simulink model "OMAP"  (R2018b)
settings: Solver=FixedStepDiscrete  StartTime=0.0  StopTime=10.0  FixedStep=0.01  RelTol=1e-3
values from neighbouring files (symbols this model uses):
  Clb_ICADirect_LaneDisp_StateFive = Simulink.Parameter    [omap_ver_442.m]
  Clb_ICADirect_LaneDisp_StateFour = Simulink.Parameter    [omap_ver_442.m]
  Clb_ICADirect_LaneDisp_StateOne = Simulink.Parameter    [omap_ver_442.m]
  Clb_ICADirect_LaneDisp_StateThree = Simulink.Parameter    [omap_ver_442.m]
  Clb_ICADirect_LaneDisp_StateTwo = Simulink.Parameter    [omap_ver_442.m]
  Clb_ICADirect_LaneDisp_StateZero = Simulink.Parameter    [omap_ver_442.m]
  Clb_ICADirect_LaneDispSW = Simulink.Parameter    [omap_ver_442.m]
  Clb_ICADirect_TrnLghtsCom_Switch = Simulink.Parameter    [omap_ver_442.m]
  Clb_ICADirect_TrnLghtsCom_Value = Simulink.Parameter    [omap_ver_442.m]
  Clb_ICADirect_TrnLghtsCrtl_Inhb = Simulink.Parameter    [omap_ver_442.m]
  OMAP_ACCAEB_EMSESC_Decel = Simulink.Parameter    [omap_ver_442.m]
  OMAP_ACCFCW_IC_Decel = Simulink.Parameter    [omap_ver_442.m]
  OMAP_clb_ACC_RVVReqType = Simulink.Parameter    [omap_ver_442.m]
  OMAP_clb_ACC_RVVReqType_Switch = Simulink.Parameter    [omap_ver_442.m]
  OMAP_clb_ACCHeadwayDisplay = Simulink.Parameter    [omap_ver_442.m]
  OMAP_clb_ACCHeadwayDisplay_Switch = Simulink.Parameter    [omap_ver_442.m]
  OMAP_clb_ACCHeadwayIcon = Simulink.Parameter    [omap_ver_442.m]
  OMAP_clb_ACCHeadwayIcon_Switch = Simulink.Parameter    [omap_ver_442.m]
  OMAP_clb_ACCMessagePrompt = Simulink.Parameter    [omap_ver_442.m]
  OMAP_clb_ACCMessagePrompt_Switch = Simulink.Parameter    [omap_ver_442.m]
  OMAP_clb_ACCRequestEPB = Simulink.Parameter    [omap_ver_442.m]
  OMAP_clb_ACCRequestEPB_Switch = Simulink.Parameter    [omap_ver_442.m]
  OMAP_clb_ACCSetSpeed = Simulink.Parameter    [omap_ver_442.m]
  OMAP_clb_ACCSetSpeed_Switch = Simulink.Parameter    [omap_ver_442.m]
  OMAP_clb_ACCSetSpeedDis = Simulink.Parameter    [omap_ver_442.m]
  OMAP_clb_ACCSetSpeedDis_Switch = Simulink.Parameter    [omap_ver_442.m]
  OMAP_clb_ACCState = Simulink.Parameter    [omap_ver_442.m]
  OMAP_clb_ACCState_Switch = Simulink.Parameter    [omap_ver_442.m]
  OMAP_clb_ACCStatusIconDis = Simulink.Parameter    [omap_ver_442.m]
  OMAP_clb_ACCStatusIconDis_Switch = Simulink.Parameter    [omap_ver_442.m]
  OMAP_clb_ACCTorqueReq = Simulink.Parameter    [omap_ver_442.m]
  OMAP_clb_ACCTorqueReq_Switch = Simulink.Parameter    [omap_ver_442.m]
  OMAP_clb_ADAS_State = Simulink.Parameter    [omap_ver_442.m]
  OMAP_clb_ADAS_State_Switch = Simulink.Parameter    [omap_ver_442.m]
  OMAP_clb_AEBAlertReq = Simulink.Parameter    [omap_ver_442.m]
  OMAP_clb_AEBAlertReq_Switch = Simulink.Parameter    [omap_ver_442.m]
  OMAP_clb_AEBBrakingProg = Simulink.Parameter    [omap_ver_442.m]
  OMAP_clb_AEBBrakingProg_Switch = Simulink.Parameter    [omap_ver_442.m]
  OMAP_clb_AEBFaultStatus = Simulink.Parameter    [omap_ver_442.m]
  OMAP_clb_AEBFaultStatus_Switch = Simulink.Parameter    [omap_ver_442.m]
  OMAP_clb_AEBMassageDisp = Simulink.Parameter    [omap_ver_442.m]
  OMAP_clb_AEBMassageDisp_Switch = Simulink.Parameter    [omap_ver_442.m]
  OMAP_clb_AEBState = Simulink.Parameter    [omap_ver_442.m]
  OMAP_clb_AEBState_Switch = Simulink.Parameter    [omap_ver_442.m]
  OMAP_clb_AEBSwitchStatus = Simulink.Parameter    [omap_ver_442.m]
  OMAP_clb_AEBSwitchStatus_Switch = Simulink.Parameter    [omap_ver_442.m]
  OMAP_clb_BrakeRequest = Simulink.Parameter    [omap_ver_442.m]
  OMAP_clb_BrakeRequest_Switch = Simulink.Parameter    [omap_ver_442.m]
  OMAP_clb_DecelerationSet = Simulink.Parameter    [omap_ver_442.m]
  OMAP_clb_DecelerationSet_Switch = Simulink.Parameter    [omap_ver_442.m]
  OMAP_clb_DecelerationType = Simulink.Parameter    [omap_ver_442.m]
  OMAP_clb_DecelerationType_Switch = Simulink.Parameter    [omap_ver_442.m]
  OMAP_clb_DeclControlReq = Simulink.Parameter    [omap_ver_442.m]
  OMAP_clb_DeclControlReq_Switch = Simulink.Parameter    [omap_ver_442.m]
  OMAP_clb_DownorUpGearMinTime = Simulink.Parameter    [omap_ver_442.m]
  OMAP_clb_DownorUpGearMinTime_Switch = Simulink.Parameter    [omap_ver_442.m]
  OMAP_clb_ELKPopupMessage = Simulink.Parameter    [omap_ver_442.m]
  OMAP_clb_ELKPopupMessage_Switch = Simulink.Parameter    [omap_ver_442.m]
  OMAP_clb_ELKSts = Simulink.Parameter    [omap_ver_442.m]
  OMAP_clb_ELKSts_Switch = Simulink.Parameter    [omap_ver_442.m]
  OMAP_clb_ESAFaultSt = Simulink.Parameter    [omap_ver_442.m]
  OMAP_clb_ESAFaultSt_Switch = Simulink.Parameter    [omap_ver_442.m]
  OMAP_clb_ESARequest = Simulink.Parameter    [omap_ver_442.m]
  OMAP_clb_ESARequest_Switch = Simulink.Parameter    [omap_ver_442.m]
  OMAP_clb_ESAState = Simulink.Parameter    [omap_ver_442.m]
  OMAP_clb_ESAState_Switch = Simulink.Parameter    [omap_ver_442.m]
  OMAP_clb_ESATorqueReq = Simulink.Parameter    [omap_ver_442.m]
  OMAP_clb_ESATorqueReq_Switch = Simulink.Parameter    [omap_ver_442.m]
  OMAP_clb_ESCDriveOff = Simulink.Parameter    [omap_ver_442.m]
  OMAP_clb_ESCDriveOff_Switch = Simulink.Parameter    [omap_ver_442.m]
  OMAP_clb_ESCHoldReq = Simulink.Parameter    [omap_ver_442.m]
  OMAP_clb_ESCHoldReq_Switch = Simulink.Parameter    [omap_ver_442.m]
  OMAP_clb_Handsoffwarning = Simulink.Parameter    [omap_ver_442.m]
  OMAP_clb_Handsoffwarning_Switch = Simulink.Parameter    [omap_ver_442.m]
  OMAP_clb_HapticAlarmReq = Simulink.Parameter    [omap_ver_442.m]
  OMAP_clb_HapticAlarmReq_Switch = Simulink.Parameter    [omap_ver_442.m]
  OMAP_clb_HMIPopupMassage = Simulink.Parameter    [omap_ver_442.m]
  OMAP_clb_HMIPopupMassage_Switch = Simulink.Parameter    [omap_ver_442.m]
  OMAP_clb_HWAActionSts = Simulink.Parameter    [omap_ver_442.m]
  OMAP_clb_HWAActionSts_Switch = Simulink.Parameter    [omap_ver_442.m]
  OMAP_clb_HWAMode = Simulink.Parameter    [omap_ver_442.m]
  OMAP_clb_HWAMode_Switch = Simulink.Parameter    [omap_ver_442.m]
  OMAP_clb_HWATurnOnIdctr = Simulink.Parameter    [omap_ver_442.m]
  OMAP_clb_HWATurnOnIdctr_Switch = Simulink.Parameter    [omap_ver_442.m]
  OMAP_clb_ICAMassageDisp = Simulink.Parameter    [omap_ver_442.m]
  OMAP_clb_ICAMassageDisp_Switch = Simulink.Parameter    [omap_ver_442.m]
  OMAP_clb_ICAStatusIcon = Simulink.Parameter    [omap_ver_442.m]
  OMAP_clb_ICAStatusIcon_Switch = Simulink.Parameter    [omap_ver_442.m]
  OMAP_clb_ISLCDriverRemind = Simulink.Parameter    [omap_ver_442.m]
  OMAP_clb_ISLCDriverRemind_Switch = Simulink.Parameter    [omap_ver_442.m]
  OMAP_clb_ISLCState = Simulink.Parameter    [omap_ver_442.m]
  OMAP_clb_ISLCState_Switch = Simulink.Parameter    [omap_ver_442.m]
  OMAP_clb_JAFaultSt = Simulink.Parameter    [omap_ver_442.m]
  OMAP_clb_JAFaultSt_Switch = Simulink.Parameter    [omap_ver_442.m]
  OMAP_clb_LCAPopupMessage = Simulink.Parameter    [omap_ver_442.m]
  OMAP_clb_LCAPopupMessage_Switch = Simulink.Parameter    [omap_ver_442.m]
  OMAP_clb_LCAStatusDisplay = Simulink.Parameter    [omap_ver_442.m]
  OMAP_clb_LCAStatusDisplay_Switch = Simulink.Parameter    [omap_ver_442.m]
  OMAP_clb_LDWStatusDisplay = Simulink.Parameter    [omap_ver_442.m]
  OMAP_clb_LDWStatusDisplay_Switch = Simulink.Parameter    [omap_ver_442.m]
  OMAP_clb_LDWWarningSt = Simulink.Parameter    [omap_ver_442.m]
  OMAP_clb_LDWWarningSt_Switch = Simulink.Parameter    [omap_ver_442.m]
  OMAP_clb_LightControlValid = Simulink.Parameter    [omap_ver_442.m]
  OMAP_clb_LightControlValid_Switch = Simulink.Parameter    [omap_ver_442.m]
  OMAP_clb_LKAActivation = Simulink.Parameter    [omap_ver_442.m]
  OMAP_clb_LKAActivation_Switch = Simulink.Parameter    [omap_ver_442.m]
  OMAP_clb_LKAAngleReq = Simulink.Parameter    [omap_ver_442.m]
  OMAP_clb_LKAAngleReq_Switch = Simulink.Parameter    [omap_ver_442.m]
  OMAP_clb_LKAMode = Simulink.Parameter    [omap_ver_442.m]
  OMAP_clb_LKAMode_Switch = Simulink.Parameter    [omap_ver_442.m]
  OMAP_clb_LKAorELK_CoolTime = Simulink.Parameter    [omap_ver_442.m]
  OMAP_clb_LKAState = Simulink.Parameter    [omap_ver_442.m]
  OMAP_clb_LKAState_Switch = Simulink.Parameter    [omap_ver_442.m]
  OMAP_clb_LKAStatusDisplay = Simulink.Parameter    [omap_ver_442.m]
  OMAP_clb_LKAStatusDisplay_Switch = Simulink.Parameter    [omap_ver_442.m]
  OMAP_clb_LKASwitchState = Simulink.Parameter    [omap_ver_442.m]
  OMAP_clb_LKASwitchState_Switch = Simulink.Parameter    [omap_ver_442.m]
  OMAP_clb_LKATorqFactReq = Simulink.Parameter    [omap_ver_442.m]
  OMAP_clb_LKATorqFactReq_Switch = Simulink.Parameter    [omap_ver_442.m]
  OMAP_clb_PrefillRequest = Simulink.Parameter    [omap_ver_442.m]
  ... (+36 more)
libraries: simulink x184, canmsglib x2
(part 9 of 14)

== system OMAP/Runnable_OMAP_10ms_sys/OMAP_Module/Subsystem/ESC_Arbitration/ACC//ICA_arb_AEB//JA ==
  note: 仲裁#3——ACC/ICA与AEB/JAEB
      | 1. 当ACC/ICA在控车且造成的实车减速度已达到（标定值暂定-2.3），若AEB只触发第一档刹车（-2），则仍以ACC/ICA优先。实时监测运算，以当前周期的实车减速度数值为准。
      | 2. 若AEB进一步触发了第二档刹车（-2以上），或者触发了JAEB刹车（总共就一档，-2以上），则AEB/JAEB根据自身的运算正常触发，无条件优先于ACC/ICA
  Input_ACCS : Inport
  Input_AEBS : Inport  Port=2
  Input_JABS : Inport  Port=3
  Input_ELKS : Inport  Port=4
  Input_IMAP : Inport  Port=5
  AEB_arb_JA : Subsystem
  Bus Creator2 : BusCreator  Inputs=8
  Bus Selector : BusSelector  OutputSignals=IMAPve_g_ESC_LonAcc_convert
  Bus Selector4 : BusSelector  OutputSignals=actuator.Function_Acc_status,actuator.OMAPve_y_ADAS_ESCDriveOff,actuator.OMAPve_y_ADAS_ESCHoldReq,actuator.MDD_deceleration_type,actuator.MDD_Decelerationcontrol_request,actuator.Deceleration_setpoint_device,actuator.OMAPve_y_ADAS_ACCRequestEPB
  Compare To Constant : simulink/Logic and Bit Operations/Compare To Constant  relop=>=  const=OMAP_ACCAEB_EMSESC_Decel  OutDataTypeStr=boolean
  Compare To Constant2 : simulink/Logic and Bit Operations/Compare To Constant  relop===  const=4  OutDataTypeStr=boolean
  Compare To Constant3 : simulink/Logic and Bit Operations/Compare To Constant  relop===  const=6  OutDataTypeStr=boolean
  Compare To Constant4 : simulink/Logic and Bit Operations/Compare To Constant  relop=~=  const=4  OutDataTypeStr=boolean
  Compare To Constant5 : simulink/Logic and Bit Operations/Compare To Constant  relop=~=  const=6  OutDataTypeStr=boolean
  Constant : Constant  Value=0  OutDataTypeStr=uint8
  Data Type Conversion1 : DataTypeConversion  OutDataTypeStr=single
  Data Type Conversion{2..5,15,17} (6 alike) : DataTypeConversion  OutDataTypeStr=uint8
  Logical Operator1 : Logic  AllPortsSameDT=off  OutDataTypeStr=boolean
  Logical Operator2 : Logic  Operator=OR  AllPortsSameDT=off  OutDataTypeStr=boolean
  Logical Operator3 : Logic  AllPortsSameDT=off  OutDataTypeStr=boolean
  Logical Operator4 : Logic  Operator=OR  AllPortsSameDT=off  OutDataTypeStr=boolean
  Logical Operator5 : Logic  AllPortsSameDT=off  OutDataTypeStr=boolean
  Switch : Switch  Criteria=u2 ~= 0
  Switch1 : Switch  Criteria=u2 ~= 0
  Out1 : Outport
  Out2 : Outport  Port=2
  tag scope: ob_isJAorDeepAEB=global, ob_isLowACCandLowAEB=global
  wires:
  Switch/1 -> Out2/1
  Data Type Conversion1/1 -> Bus Creator2/7  "OMAPve_g_Deceleration_setpoint_device_1"
  Input_ACCS/1 -> Bus Selector4/1
  Constant/1 -> Bus Creator2/4  "OMAPve_y_AEB_Braking_progress_1"
  Data Type Conversion3/1 -> Bus Creator2/5  "OMAPve_y_Decel_Request_1"
  Bus Selector4/5 -> Data Type Conversion15/1, Data Type Conversion3/1  "<MDD_Decelerationcontrol_request>"
  Data Type Conversion17/1 -> Bus Creator2/3  "OMAPve_y_MDD_deceleration_type_1"
  Data Type Conversion15/1 -> Bus Creator2/6  "OMAPve_y_MDD_Decelerationcontrol_request_1"
  Bus Selector/1 -> Compare To Constant/1  "<IMAPve_g_ESC_LonAcc_convert>"
  Bus Selector4/4 -> Data Type Conversion17/1  "<MDD_deceleration_type>"
  Switch1/1 -> Switch/3
  Bus Creator2/1 -> Switch1/3
  AEB_arb_JA/2(Out2) -> Switch1/1, Switch/1
  Input_AEBS/1 -> AEB_arb_JA/1(Input_AEBS)
  Input_JABS/1 -> AEB_arb_JA/2(Input_JABS)
  AEB_arb_JA/1(Out1) -> Out1/1
  Input_IMAP/1 -> Bus Selector/1
  Logical Operator2/1 -> Logical Operator1/2
  Logical Operator5/1 -> Logical Operator2/1
  Bus Selector4/6 -> Data Type Conversion1/1  "<Deceleration_setpoint_device>"
  Logical Operator3/1 -> Logical Operator2/2
  Logical Operator4/1 -> Logical Operator3/1
  AEB_arb_JA/4(Out4) -> Logical Operator1/1
  Compare To Constant/1 -> Logical Operator3/2
  Bus Selector4/1 -> Compare To Constant4/1, Compare To Constant5/1, Compare To Constant2/1, Compare To Constant3/1  "<Function_Acc_status>"
  Compare To Constant2/1 -> Logical Operator4/1
  Compare To Constant3/1 -> Logical Operator4/2
  Compare To Constant4/1 -> Logical Operator5/1
  Compare To Constant5/1 -> Logical Operator5/2
  Input_ELKS/1 -> AEB_arb_JA/3(Input_ELKS)
  Data Type Conversion2/1 -> Bus Creator2/2  "OMAPve_y_ADAS_ESCHoldReq"
  Data Type Conversion4/1 -> Bus Creator2/1  "OMAPve_y_ADAS_ESCDriveOff"
  Bus Selector4/2 -> Data Type Conversion4/1  "<OMAPve_y_ADAS_ESCDriveOff>"
  Bus Selector4/3 -> Data Type Conversion2/1  "<OMAPve_y_ADAS_ESCHoldReq>"
  Bus Selector4/7 -> Data Type Conversion5/1  "<OMAPve_y_ADAS_ACCRequestEPB>"
  Data Type Conversion5/1 -> Bus Creator2/8  "OMAPve_y_ADAS_ACCRequestEPB"
  Logical Operator1/1 -> [ob_isLowACCandLowAEB], Switch1/2
  AEB_arb_JA/3(Out3) -> [ob_isJAorDeepAEB], Switch/2

== system OMAP/Runnable_OMAP_10ms_sys/OMAP_Module/Subsystem/ESC_Arbitration/FAPA_arb_ADAS ==
  note: 仲裁#21——FAPA与ADAS
      | 1. 关于EMS、ESC、EPS执行器控制：FAPA在控制车辆的工作阶段，无条件优先于ADAS各个功能；在其他情况，则直连ADAS内部原本的仲裁结果
      | 2. 关于仪表显示：维持原本的仲裁策略
      | 3. 选用的表征信号，经IMAP转译后为IMAPve_d_APA_AutoPark_WorkSt
  Input_ACCICAAEBJA1 : Inport
  Input_ACCICAAEBJA2 : Inport  Port=2
  Input_FAPA : Inport  Port=3
  Bus Creator5 : BusCreator  Inputs=13
  Bus Creator6 : BusCreator  Inputs=13
  Bus Selector : BusSelector  OutputSignals=OMAPve_y_ADAS_ESCDriveOff,OMAPve_y_ADAS_ESCHoldReq,OMAPve_g_Deceleration_setpoint_device_1,OMAPve_y_MDD_Decelerationcontrol_request_1,OMAPve_y_MDD_deceleration_type_1,OMAPve_y_Decel_Request_1,OMAPve_y_AEB_Braking_progress_1,OMAPve_y_ADAS_ACCRequestEPB
  Bus Selector1 : BusSelector  OutputSignals=OMAPve_y_FCW_Status_1,OMAPve_y_State_of_the_functionFARC_det_1,OMAPve_y_AEB_Status_1,OMAPve_y_Prefill_request_1,OMAPve_y_Haptic_Alarm_1
  Bus Selector2 : BusSelector  OutputSignals=IMAPve_d_APA_AutoPark_WorkSt
  Data Type Conversion{6,8..9,12..13} (5 alike) : DataTypeConversion  OutDataTypeStr=uint8
  OMAPve_g_Deceleration_setpoint_deviceNum : Constant  Value=2.05  OutDataTypeStr=single
  OMAPve_y_ADAS_ACCRequestEPBNum : Constant  Value=0  OutDataTypeStr=uint8
  OMAPve_y_ADAS_ESCDriveOffNum : Constant  Value=0  OutDataTypeStr=uint8
  OMAPve_y_ADAS_ESCHoldReqNum : Constant  Value=0  OutDataTypeStr=uint8
  OMAPve_y_AEB_Braking_progressNum : Constant  Value=0  OutDataTypeStr=uint8
  OMAPve_y_AEB_StatusNum : Constant  Value=0  OutDataTypeStr=uint8
  OMAPve_y_Decel_RequestNum : Constant  Value=0  OutDataTypeStr=uint8
  OMAPve_y_FCW_StatusNum : Constant  Value=10  OutDataTypeStr=uint8
  OMAPve_y_Haptic_AlarmNum : Constant  Value=0  OutDataTypeStr=uint8
  OMAPve_y_MDD_Decelerationcontrol_requestNum : Constant  Value=0  OutDataTypeStr=uint8
  OMAPve_y_MDD_deceleration_typeNum : Constant  Value=0  OutDataTypeStr=uint8
  OMAPve_y_Prefill_requestNum : Constant  Value=0  OutDataTypeStr=uint8
  OMAPve_y_State_of_the_functionFARC_detNum : Constant  Value=0  OutDataTypeStr=uint8
  Switch : Switch  Criteria=u2 ~= 0
  Arbitration_ESC : Outport
  wires:
  OMAPve_y_State_of_the_functionFARC_detNum/1 -> Bus Creator5/2  "OMAPve_y_State_of_the_functionFARC_det_1"
  OMAPve_y_Decel_RequestNum/1 -> Bus Creator5/11  "OMAPve_y_Decel_Request_1"
  OMAPve_y_MDD_deceleration_typeNum/1 -> Bus Creator5/10  "OMAPve_y_MDD_deceleration_type_1"
  Bus Creator5/1 -> Switch/1  "LKA_ESC"
  Data Type Conversion6/1 -> Bus Creator6/4  "OMAPve_y_Prefill_request_1"
  Data Type Conversion8/1 -> Bus Creator6/2  "OMAPve_y_State_of_the_functionFARC_det_1"
  OMAPve_y_Prefill_requestNum/1 -> Bus Creator5/4  "OMAPve_y_Prefill_request_1"
  Data Type Conversion13/1 -> Bus Creator6/5  "OMAPve_y_Haptic_Alarm_1"
  OMAPve_g_Deceleration_setpoint_deviceNum/1 -> Bus Creator5/8  "OMAPve_g_Deceleration_setpoint_device_1"
  OMAPve_y_AEB_StatusNum/1 -> Bus Creator5/3  "OMAPve_y_AEB_Status_1"
  OMAPve_y_FCW_StatusNum/1 -> Bus Creator5/1  "OMAPve_y_FCW_Status_1"
  Bus Selector/8 -> Bus Creator6/13  "<OMAPve_y_ADAS_ACCRequestEPB>"
  OMAPve_y_ADAS_ACCRequestEPBNum/1 -> Bus Creator5/13  "OMAPve_y_ADAS_ACCRequestEPB"
  OMAPve_y_ADAS_ESCDriveOffNum/1 -> Bus Creator5/6  "OMAPve_y_ADAS_ESCDriveOff"
  Bus Selector1/5 -> Data Type Conversion13/1  "<OMAPve_y_Haptic_Alarm_1>"
  Bus Selector2/1 -> Switch/2  "<IMAPve_d_APA_AutoPark_WorkSt>"
  OMAPve_y_MDD_Decelerationcontrol_requestNum/1 -> Bus Creator5/9  "OMAPve_y_MDD_Decelerationcontrol_request_1"
  Data Type Conversion9/1 -> Bus Creator6/3  "OMAPve_y_AEB_Status_1"
  OMAPve_y_AEB_Braking_progressNum/1 -> Bus Creator5/12  "OMAPve_y_AEB_Braking_progress_1"
  OMAPve_y_Haptic_AlarmNum/1 -> Bus Creator5/5  "OMAPve_y_Haptic_Alarm_1"
  OMAPve_y_ADAS_ESCHoldReqNum/1 -> Bus Creator5/7  "OMAPve_y_ADAS_ESCHoldReq"
  Bus Creator6/1 -> Switch/3  "Arbitration_ESC"
  Bus Selector/3 -> Bus Creator6/8  "<OMAPve_g_Deceleration_setpoint_device_1>"
  Bus Selector/7 -> Bus Creator6/12  "<OMAPve_y_AEB_Braking_progress_1>"
  Bus Selector/6 -> Bus Creator6/11  "<OMAPve_y_Decel_Request_1>"
  Data Type Conversion12/1 -> Bus Creator6/1  "OMAPve_y_FCW_Status_1"
  Bus Selector1/4 -> Data Type Conversion6/1  "<OMAPve_y_Prefill_request_1>"
  Bus Selector1/1 -> Data Type Conversion12/1  "<OMAPve_y_FCW_Status_1>"
  Input_ACCICAAEBJA1/1 -> Bus Selector1/1
  Bus Selector1/3 -> Data Type Conversion9/1  "<OMAPve_y_AEB_Status_1>"
  Bus Selector/4 -> Bus Creator6/9  "<OMAPve_y_MDD_Decelerationcontrol_request_1>"
  Bus Selector1/2 -> Data Type Conversion8/1  "<OMAPve_y_State_of_the_functionFARC_det_1>"
  Input_ACCICAAEBJA2/1 -> Bus Selector/1
  Bus Selector/1 -> Bus Creator6/6  "<OMAPve_y_ADAS_ESCDriveOff>"
  Bus Selector/5 -> Bus Creator6/10  "<OMAPve_y_MDD_deceleration_type_1>"
  Bus Selector/2 -> Bus Creator6/7  "<OMAPve_y_ADAS_ESCHoldReq>"
  Switch/1 -> Arbitration_ESC/1  "Arbitration_ESC"
  Input_FAPA/1 -> Bus Selector2/1

== system OMAP/Runnable_OMAP_10ms_sys/OMAP_Module/Subsystem/IC_Arbitration/ACC//ICA_arb_FCW//JACW ==
  note: 仲裁#2——ACC/ICA与FCW/JACW
      | 1. ACC/ICA算出的期望减速度>（标定值）时，FCW强制不触发
      | 2. 否则，FCW/JACW根据自身的运算正常触发
  Input_ACCS : Inport
  <AEBSve_d_AEBAlertReq_convert> : Inport  Port=2
  Compare To Constant : simulink/Logic and Bit Operations/Compare To Constant  relop=<=  const=OMAP_ACCFCW_IC_Decel  OutDataTypeStr=boolean
  Compare To Constant1 : simulink/Logic and Bit Operations/Compare To Constant  relop===  const=1  OutDataTypeStr=boolean
  Compare To Zero : simulink/Logic and Bit Operations/Compare To Zero  relop=>=  OutDataTypeStr=boolean
  Logical Operator1 : Logic  Operator=OR  AllPortsSameDT=off  OutDataTypeStr=boolean
  Switch : Switch  Criteria=u2 ~= 0  OutDataTypeStr=uint8
  Out1 : Outport
  wires:
  Compare To Constant1/1 -> Switch/2
  Compare To Constant/1 -> Logical Operator1/2
  Switch/1 -> Out1/1
  Logical Operator1/1 -> Switch/1
  Compare To Zero/1 -> Logical Operator1/1
  Input_ACCS/1 -> Compare To Zero/1, Compare To Constant/1
  <AEBSve_d_AEBAlertReq_convert>/1 -> Switch/3, Compare To Constant1/1

== system OMAP/Runnable_OMAP_10ms_sys/OMAP_Module/Subsystem/IC_Arbitration/ACC_ICA ==
  ACC_Message : Inport
  ICA_Message : Inport  Port=2
  MATLAB Function : MATLAB Function  TreatAsAtomicUnit=on
  ACC_Message_out : Outport
  ICA_Message_out : Outport  Port=2
  wires:
  ACC_Message/1 -> MATLAB Function/1(ACC_Message)
  ICA_Message/1 -> MATLAB Function/2(ICA_Message)
  MATLAB Function/1(ACC_Message_out) -> ACC_Message_out/1
  MATLAB Function/2(ICA_Message_out) -> ICA_Message_out/1

== system OMAP/Runnable_OMAP_10ms_sys/OMAP_Module/Subsystem/IC_Arbitration/AEB//JA_arb_ELK ==
  note: 仲裁#8——AEB/FCW/JAEB/JACW与ELK
      | 1.AEB/FCW/JAEB/JACW无条件优先于ELK
  Input_AEBS : Inport
  Input_JABS : Inport  Port=2
  Input_ELKS : Inport  Port=3
  Bus Creator : BusCreator  Inputs=5
  Bus Selector : BusSelector  OutputSignals=AEBSve_d_AEBAlertReq_convert
  Bus Selector2 : BusSelector  OutputSignals=ELKSve_y_Hands_Off_Warning_convert,ELKSve_y_ELK_VehicleLaneDisp_convert,ELKSve_y_ELK_Action_Indication_convert,ELKSve_y_ELK_ELKSts_convert,ELKSve_y_EPS_State_Control_convert
  Bus Selector3 : BusSelector  OutputSignals=JABSve_d_DbAlertReq_convert
  Compare To Constant : simulink/Logic and Bit Operations/Compare To Constant  relop=~=  const=0  OutDataTypeStr=boolean
  Compare To Constant1 : simulink/Logic and Bit Operations/Compare To Constant  relop=~=  const=0  OutDataTypeStr=boolean
  Data Type Conversion{1..5} (5 alike) : DataTypeConversion  OutDataTypeStr=uint8
  Index Vector{1..5} (5 alike) : MultiPortSwitch  DataPortOrder=Zero-based contiguous  Inputs=2  zeroidx=on  OutDataTypeStr=uint8
  Logical Operator : Logic  Operator=OR  AllPortsSameDT=off  OutDataTypeStr=boolean
  OMAPve_y_ADAS_ELKStsNum1 : Constant  Value=0  OutDataTypeStr=uint8
  OMAPve_y_General_state_of_LKA_function3F2Num : Constant  Value=0  OutDataTypeStr=uint8
  OMAPve_y_Hands_off_warningNum : Constant  Value=0  OutDataTypeStr=uint8
  OMAPve_y_LKA_action_indicationNum : Constant  Value=0  OutDataTypeStr=uint8
  OMAPve_y_Vehicle_Lane_DisplayNum : Constant  Value=0  OutDataTypeStr=uint8
  Out1 : Outport
  wires:
  Input_JABS/1 -> Bus Selector3/1
  Bus Selector3/1 -> Compare To Constant1/1  "<JABSve_d_DbAlertReq_convert>"
  Compare To Constant1/1 -> Logical Operator/2
  Bus Selector/1 -> Compare To Constant/1  "<AEBSve_d_AEBAlertReq_convert>"
  Input_AEBS/1 -> Bus Selector/1
  Compare To Constant/1 -> Logical Operator/1
  Bus Creator/1 -> Out1/1
  Input_ELKS/1 -> Bus Selector2/1
  Bus Selector2/1 -> Index Vector5/2  "<ELKSve_y_Hands_Off_Warning_convert>"
  OMAPve_y_Hands_off_warningNum/1 -> Index Vector5/3  "OMAPve_y_Hands_off_warning_2"
  Index Vector5/1 -> Data Type Conversion5/1
  Data Type Conversion5/1 -> Bus Creator/1  "OMAPve_y_Hands_off_warning_2"
  Bus Selector2/3 -> Index Vector1/2  "<ELKSve_y_ELK_Action_Indication_convert>"
  Data Type Conversion1/1 -> Bus Creator/3  "OMAPve_y_LKA_action_indication_2"
  Index Vector1/1 -> Data Type Conversion1/1
  OMAPve_y_LKA_action_indicationNum/1 -> Index Vector1/3  "OMAPve_y_LKA_action_indication_2"
  Bus Selector2/4 -> Index Vector2/2  "<ELKSve_y_ELK_ELKSts_convert>"
  Data Type Conversion2/1 -> Bus Creator/4  "OMAPve_y_ADAS_ELKSts_2"
  Index Vector2/1 -> Data Type Conversion2/1
  OMAPve_y_ADAS_ELKStsNum1/1 -> Index Vector2/3  "OMAPve_y_ADAS_ELKSts_2"
  Index Vector3/1 -> Data Type Conversion3/1
  OMAPve_y_Vehicle_Lane_DisplayNum/1 -> Index Vector3/3  "OMAPve_y_Vehicle_Lane_Display_2"
  Bus Selector2/2 -> Index Vector3/2  "<ELKSve_y_ELK_VehicleLaneDisp_convert>"
  Logical Operator/1 -> Index Vector4/1, Index Vector2/1, Index Vector1/1, Index Vector3/1, Index Vector5/1
  Data Type Conversion3/1 -> Bus Creator/2  "OMAPve_y_Vehicle_Lane_Display_2"
  Bus Selector2/5 -> Index Vector4/2  "<ELKSve_y_EPS_State_Control_convert>"
  OMAPve_y_General_state_of_LKA_function3F2Num/1 -> Index Vector4/3  "OMAPve_y_General_state_of_LKA_function3F2_2"
  Index Vector4/1 -> Data Type Conversion4/1
  Data Type Conversion4/1 -> Bus Creator/5  "OMAPve_y_General_state_of_LKA_function3F2_2"

== system OMAP/Runnable_OMAP_10ms_sys/OMAP_Module/Subsystem/IC_Arbitration/AEB_arb_JA ==
  note: 仲裁#22——AEB/FCW与JAEB/JACW
      | alert优先级：AEB > JAEB > JACW > FCW。若新出现了更高优先级的，则随时覆盖；被覆盖的更低优先级的，不再另计时
  Input_AEBS : Inport
  Input_JABS : Inport  Port=2
  Bus Creator : BusCreator  Inputs=5
  Bus Selector3 : BusSelector  OutputSignals=JABSve_d_DbAlertReq_convert,JABSve_d_DbFltStatus_convert,JABSve_d_DbSwitchStatus_convert,JABSve_d_DbTips_convert
  Bus Selector4 : BusSelector  OutputSignals=AEBSve_d_AEBAlertReq_convert,AEBSve_d_AEBFaultStatus_convert,AEBSve_d_AEBSwitchStatus_convert,AEBSve_d_AEBTips_convert
  Data Type Conversion{1,12..15} (5 alike) : DataTypeConversion  OutDataTypeStr=uint8
  Subsystem : Subsystem
  Terminator : Terminator
  Terminator1 : Terminator
  Out1 : Outport
  wires:
  Data Type Conversion13/1 -> Bus Creator/2  "OMAPve_y_AEB_Fault_Status_2"
  Input_JABS/1 -> Bus Selector3/1
  Data Type Conversion12/1 -> Bus Creator/1  "OMAPve_y_AEB_Alert_Req_2"
  Bus Selector3/4 -> Terminator1/1  "<JABSve_d_DbTips_convert>"
  Bus Selector4/2 -> Data Type Conversion13/1  "<AEBSve_d_AEBFaultStatus_convert>"
  Data Type Conversion15/1 -> Bus Creator/4  "OMAPve_y_AEB_tips_2"
  Data Type Conversion14/1 -> Bus Creator/3  "OMAPve_y_AEB_Switch_Status_2"
  Bus Selector3/3 -> Terminator/1  "<JABSve_d_DbSwitchStatus_convert>"
  Bus Selector4/3 -> Data Type Conversion14/1  "<AEBSve_d_AEBSwitchStatus_convert>"
  Bus Selector4/4 -> Data Type Conversion15/1  "<AEBSve_d_AEBTips_convert>"
  Bus Creator/1 -> Out1/1
  Bus Selector3/2 -> Data Type Conversion1/1  "<JABSve_d_DbFltStatus_convert>"
  Input_AEBS/1 -> Bus Selector4/1
  Data Type Conversion1/1 -> Bus Creator/5  "OMAPve_y_ADAS_JAFaultSt_2"
  Bus Selector4/1 -> Subsystem/1(<AEBSve_d_AEBAlertReq_convert>)  "<AEBSve_d_AEBAlertReq_convert>"
  Bus Selector3/1 -> Subsystem/2(<JABSve_d_DbAlertReq_convert>)  "<JABSve_d_DbAlertReq_convert>"
  Subsystem/1(Out1) -> Data Type Conversion12/1

== system OMAP/Runnable_OMAP_10ms_sys/OMAP_Module/Subsystem/IC_Arbitration/ICA_arb_LKA//ELK ==
  note: 仲裁#23——ICA与LKA/LDW/ELK
      | ICA与LKA和ELK的仲裁，关于HMI：
      | 1. 脱手报警（声音）——ICA_STATE为3期间独占脱手报警；ICA_STATE为4期间，取ICA脱手报警 或 LKA/ELK脱手报警；其他情况，取LKA/ELK脱手报警
      | 2. 车道线涂色——ICA_STATE不为3且LKA/ELK的lane_display不为0则LKA/ELK优先，否则ICA优先
  Input_ICA : Inport
  Input_LKAELK : Inport  Port=2
  Bus Creator : BusCreator  Inputs=4
  Bus Selector : BusSelector  OutputSignals=OMAPve_y_Vehicle_Lane_Display_2,OMAPve_y_Hands_off_warning_2,OMAPve_y_HMI_Popup_Status_2
  Bus Selector3 : BusSelector  OutputSignals=HMI.OMAPve_y_ICA_HMI_Txt_Disp_2,HMI.OMAPve_y_Vehicle_Lane_Display_2,actuator.ICABve_d_ICAState_convert,HMI.OMAPve_y_Hands_off_warning_2
  Compare To Constant : simulink/Logic and Bit Operations/Compare To Constant  relop=~=  const=3.0  OutDataTypeStr=boolean
  Compare To Constant1 : simulink/Logic and Bit Operations/Compare To Constant  relop=~=  const=0  OutDataTypeStr=boolean
  Data Type Conversion2 : DataTypeConversion  OutDataTypeStr=uint8
  Index Vector1 : MultiPortSwitch  DataPortOrder=Zero-based contiguous  Inputs=6  zeroidx=on  OutDataTypeStr=uint8
  Logical Operator1 : Logic  Operator=OR  AllPortsSameDT=off  OutDataTypeStr=boolean
  Logical Operator2 : Logic  AllPortsSameDT=off  OutDataTypeStr=boolean
  Switch1 : Switch  Criteria=u2 ~= 0  OutDataTypeStr=uint8
  Out1 : Outport
  wires:
  Bus Creator/1 -> Out1/1
  Bus Selector3/3 -> Compare To Constant/1, Index Vector1/1  "<ICABve_d_ICAState_convert>"
  Input_ICA/1 -> Bus Selector3/1
  Bus Selector3/4 -> Index Vector1/5, Logical Operator1/1  "<OMAPve_y_Hands_off_warning_2>"
  Index Vector1/1 -> Bus Creator/3  "OMAPve_y_Hands_off_warning_2"
  Switch1/1 -> Bus Creator/2  "OMAPve_y_Vehicle_Lane_Display_2"
  Input_LKAELK/1 -> Bus Selector/1
  Bus Selector/2 -> Index Vector1/2, Index Vector1/3, Index Vector1/4, Index Vector1/7, Logical Operator1/2  "<OMAPve_y_Hands_off_warning_2>"
  Data Type Conversion2/1 -> Bus Creator/1  "OMAPve_y_ICA_HMI_Txt_Disp_2"
  Bus Selector3/1 -> Data Type Conversion2/1  "<OMAPve_y_ICA_HMI_Txt_Disp_2>"
  Bus Selector/3 -> Bus Creator/4  "<OMAPve_y_HMI_Popup_Status_2>"
  Bus Selector/1 -> Switch1/1, Compare To Constant1/1  "<OMAPve_y_Vehicle_Lane_Display_2>"
  Bus Selector3/2 -> Switch1/3  "<OMAPve_y_Vehicle_Lane_Display_2>"
  Logical Operator1/1 -> Index Vector1/6
  Compare To Constant/1 -> Logical Operator2/1
  Compare To Constant1/1 -> Logical Operator2/2
  Logical Operator2/1 -> Switch1/2

== system OMAP/Runnable_OMAP_10ms_sys/OMAP_Module/Subsystem/IC_Arbitration/LKA_arb_ELK ==
  note: 仲裁#7——ELK与LKA
      | ELK开关关闭时输出LKA；ELK开关打开时：1、对EPS和车道线显示：默认输出LKA，谁先发出控制指令上升沿便输出谁，直到该功能控制指令消失的标定时间后再重新根据谁先发出控制指令的上升沿来判断输出谁，在标定时间内被输出功能若再次出现控制指令上升沿，则再次响应输出该功能；2、对脱手报警：对LKA与ELK的脱手报警取或
  Input_FDMM : Inport
  Input_LKAS : Inport  Port=2
  Input_ELKS : Inport  Port=3
  AND : Logic  AllPortsSameDT=off  OutDataTypeStr=boolean
  Bus Creator1 : BusCreator  Inputs=9
  Bus Selector : BusSelector  OutputSignals=LKASve_y_HMI_Popup_Status_convert,LKASve_y_Hands_Off_Warning_convert,LKASve_y_Vehicle_Lane_Display_convert,LKASve_y_LDW_Flag_convert,LKASve_y_LDW_Status_Display_convert,LKASve_y_LKA_Status_Display_convert,LKASve_y_LKA_Action_Indication_convert,LKASve_y_EPS_State_Control_convert
  Bus Selector1 : BusSelector  OutputSignals=OMAPve_y_Hands_off_warning_2,OMAPve_y_Vehicle_Lane_Display_2,OMAPve_y_LKA_action_indication_2,OMAPve_y_General_state_of_LKA_function3F2_2,OMAPve_y_ADAS_ELKSts_2
  Bus Selector2 : BusSelector  OutputSignals=FDMMve_d_ElkFcnConf_convert,FDMMve_d_LkaFcnConf_convert
  Compare To Constant : simulink/Logic and Bit Operations/Compare To Constant  relop===  const=uint16(0)  OutDataTypeStr=boolean
  Compare To Constant1 : simulink/Logic and Bit Operations/Compare To Constant  relop===  const=uint16(1)  OutDataTypeStr=boolean
  Data Type Conversion{1..3,5,7..11} (9 alike) : DataTypeConversion  OutDataTypeStr=uint8
  Ground : Ground
  Ground1 : Ground
  Index Vector{1..2,6..8} (5 alike) : MultiPortSwitch  Inputs=2  OutDataTypeStr=uint8
  Index Vector{3..5,9..10} (5 alike) : MultiPortSwitch  DataPortOrder=Zero-based contiguous  Inputs=2  zeroidx=on  OutDataTypeStr=uint8
  OR : Logic  Operator=OR  AllPortsSameDT=off  OutDataTypeStr=boolean
  Subsystem : Subsystem
  Out1 : Outport
  wires:
  Input_LKAS/1 -> Bus Selector/1
  Input_ELKS/1 -> Bus Selector1/1
  Data Type Conversion5/1 -> Bus Creator1/2  "OMAPve_y_Hands_off_warning_2"
  Data Type Conversion9/1 -> Bus Creator1/5  "OMAPve_y_LDW_Status_Display_2"
  Data Type Conversion7/1 -> Bus Creator1/3  "OMAPve_y_Vehicle_Lane_Display_2"
  Data Type Conversion10/1 -> Bus Creator1/6  "OMAPve_y_LKA_Status_Display_2"
  Data Type Conversion8/1 -> Bus Creator1/4  "OMAPve_y_LDW_Flag_2"
  Bus Creator1/1 -> Out1/1
  OR/1 -> Data Type Conversion5/1
  Data Type Conversion11/1 -> Bus Creator1/7  "OMAPve_y_LKA_action_indication_2"
  Index Vector3/1 -> Data Type Conversion7/1
  Index Vector4/1 -> Data Type Conversion8/1
  Index Vector5/1 -> Data Type Conversion9/1
  Bus Selector/2 -> OR/1  "<LKASve_y_Hands_Off_Warning_convert>"
  Bus Selector/3 -> Index Vector6/2  "<LKASve_y_Vehicle_Lane_Display_convert>"
  Bus Selector/4 -> Index Vector7/2  "<LKASve_y_LDW_Flag_convert>"
  Bus Selector/5 -> Index Vector8/2  "<LKASve_y_LDW_Status_Display_convert>"
  Bus Selector/7 -> Index Vector1/2  "<LKASve_y_LKA_Action_Indication_convert>"
  Bus Selector1/1 -> OR/2  "<OMAPve_y_Hands_off_warning_2>"
  Ground/1 -> Index Vector4/3, Index Vector7/3
  Ground1/1 -> Index Vector5/3, Index Vector8/3
  Bus Selector1/3 -> Index Vector9/3, Index Vector1/3  "<OMAPve_y_LKA_action_indication_2>"
  Index Vector9/1 -> Data Type Conversion11/1
  Data Type Conversion1/1 -> Bus Creator1/9  "OMAPve_y_ADAS_ELKSts_2"
  Bus Selector1/5 -> Data Type Conversion1/1  "<OMAPve_y_ADAS_ELKSts_2>"
  Bus Selector1/2 -> Index Vector3/3, Index Vector6/3  "<OMAPve_y_Vehicle_Lane_Display_2>"
  Bus Selector/1 -> Data Type Conversion2/1  "<LKASve_y_HMI_Popup_Status_convert>"
  Data Type Conversion2/1 -> Bus Creator1/1  "OMAPve_y_HMI_Popup_Status_2"
  Data Type Conversion3/1 -> Bus Creator1/8  "OMAPve_y_General_state_of_LKA_function3F2_2"
  Index Vector10/1 -> Data Type Conversion3/1
  Bus Selector/8 -> Subsystem/1(<LKASve_y_EPS_State_Control_convert>), Index Vector2/2  "<LKASve_y_EPS_State_Control_convert>"
  Bus Selector1/4 -> Subsystem/2(<OMAPve_y_General_state_of_LKA_function3F2_2>), Index Vector10/3, Index Vector2/3  "<OMAPve_y_General_state_of_LKA_function3F2_2>"
  Bus Selector/6 -> Data Type Conversion10/1  "<LKASve_y_LKA_Status_Display_convert>"
  Input_FDMM/1 -> Bus Selector2/1
  Index Vector6/1 -> Index Vector3/2
  Index Vector7/1 -> Index Vector4/2
  Index Vector8/1 -> Index Vector5/2
  Index Vector1/1 -> Index Vector9/2
  Index Vector2/1 -> Index Vector10/2
  Subsystem/1(state) -> Index Vector7/1, Index Vector8/1, Index Vector1/1, Index Vector2/1, Index Vector6/1
  Bus Selector2/2 -> Compare To Constant/1  "<FDMMve_d_LkaFcnConf_convert>"
  Bus Selector2/1 -> Compare To Constant1/1  "<FDMMve_d_ElkFcnConf_convert>"
  Compare To Constant1/1 -> AND/1
  Compare To Constant/1 -> AND/2
  AND/1 -> Index Vector3/1, Index Vector10/1, Index Vector9/1, Index Vector5/1, Index Vector4/1

== system OMAP/Runnable_OMAP_10ms_sys/OMAP_Module/ACCS_Direct/ACCS_Define/ACC_State_Synthesis(ACC_SS)/If Action Subsystem2 ==
  In1 : Inport
  Action Port : ActionPort  InitializeStates=reset  ActionType=then
  Bus Creator : BusCreator  Inputs=15
  Constant : Constant  Value=2.05  OutDataTypeStr=single
  Constant1 : Constant  Value=6.2  OutDataTypeStr=single
  Constant{3,5,7,9..10} (5 alike) : Constant  Value=0  OutDataTypeStr=uint8
  Constant2 : Constant  Value=6.2  OutDataTypeStr=single
  Constant4 : Constant  Value=-4000  OutDataTypeStr=single
  Constant6 : Constant  Value=-4000  OutDataTypeStr=single
  OMAPve_y_ADAS_ACCRequestEPBNum1 : Constant  Value=0  OutDataTypeStr=uint8
  OMAPve_y_ADAS_ESCDriveOffNum : Constant  Value=0  OutDataTypeStr=uint8
  OMAPve_y_ADAS_ESCHoldReq : Constant  Value=0  OutDataTypeStr=uint8
  Signal Conversion : SignalConversion  OverrideOpt=off
  Subsystem : Subsystem
  Subsystem4 : Subsystem
  Control_Ouput : Outport
  wires:
  Signal Conversion/1 -> Control_Ouput/1
  Constant5/1 -> Bus Creator/12  "Power_steering_power_cut3F2"
  Bus Creator/1 -> Signal Conversion/1
  Subsystem/1(Function_Acc_status) -> Bus Creator/6  "Function_Acc_status"
  In1/1 -> Subsystem/1(In1)
  Constant10/1 -> Bus Creator/11  "MDD_deceleration_type"
  Constant9/1 -> Bus Creator/10  "MDD_Decelerationcontrol_request"
  Subsystem4/1(TYPE_RAPPORT) -> Bus Creator/9  "TYPE_RAPPORT"
  Constant7/1 -> Bus Creator/8  "Powertrain_torquewheel_request"
  Constant6/1 -> Bus Creator/7  "ACCTqReq"
  Constant4/1 -> Bus Creator/5  "PotACCTqReq"
  Constant3/1 -> Bus Creator/4  "StAcvTqWhlPTPotReq"
  Constant2/1 -> Bus Creator/3  "TminUpGear"
  Constant1/1 -> Bus Creator/2  "TminDownGear"
  Constant/1 -> Bus Creator/1  "Deceleration_setpoint_device"
  OMAPve_y_ADAS_ESCDriveOffNum/1 -> Bus Creator/13  "OMAPve_y_ADAS_ESCDriveOff"
  OMAPve_y_ADAS_ESCHoldReq/1 -> Bus Creator/14  "OMAPve_y_ADAS_ESCHoldReq"
  OMAPve_y_ADAS_ACCRequestEPBNum1/1 -> Bus Creator/15  "OMAPve_y_ADAS_ACCRequestEPB"

== system OMAP/Runnable_OMAP_10ms_sys/OMAP_Module/ACCS_Direct/ACCS_Define/ACC_State_Synthesis(ACC_SS)/If Action Subsystem3 ==
  ACT_Control_Signal : Inport
  Action Port : ActionPort  InitializeStates=reset  ActionType=else
  Bus Creator : BusCreator  Inputs=15
  Bus Selector1 : BusSelector  OutputSignals=ACCSve_g_ACC_TqReq_convert,ACCSve_d_ACC_TqFlag_convert,ACCSve_g_ACC_DecReq_convert,ACCSve_d_ACC_DecFlag_convert,ACCSve_d_ACC_State_convert,ACCSve_d_ACC_ESCDriveOff_convert,ACCSve_d_ACC_ESCHoldReq_convert,ACCSve_d_ACC_EPBReq_convert
  Constant5 : Constant  Value=0  OutDataTypeStr=uint8
  Data Type Conversion{,1..6} (7 alike) : DataTypeConversion  OutDataTypeStr=uint8
  Gain : Gain  OutDataTypeStr=single
  Signal Conversion : SignalConversion  OverrideOpt=off
  Subsystem : Subsystem
  Subsystem1 : Subsystem
  Subsystem2 : Subsystem
  Subsystem3 : Subsystem
  Subsystem5 : Subsystem
  Subsystem6 : Subsystem
  Control_Ouput : Outport
  wires:
  Bus Selector1/4 -> [ESC_Enable]  "<ACCSve_d_ACC_DecFlag_convert>"
  Bus Selector1/3 -> [ESC_DecTar]  "<ACCSve_g_ACC_DecReq_convert>"
  Bus Selector1/2 -> [EMS_Enable]  "<ACCSve_d_ACC_TqFlag_convert>"
  Bus Selector1/1 -> [EMS_DecTar]  "<ACCSve_g_ACC_TqReq_convert>"
  Data Type Conversion2/1 -> Bus Creator/11  "MDD_deceleration_type"
  Data Type Conversion1/1 -> Bus Creator/10  "MDD_Decelerationcontrol_request"
  Data Type Conversion/1 -> Bus Creator/8  "Powertrain_torquewheel_request"
  Subsystem6/1(TYPE_RAPPORT) -> Bus Creator/9  "TYPE_RAPPORT"
  [EMS_Enable] -> Data Type Conversion/1
  Signal Conversion/1 -> Control_Ouput/1
  Constant5/1 -> Bus Creator/12  "Power_steering_power_cut3F2"
  Gain/1 -> Bus Creator/5  "PotACCTqReq"
  [EMS_Enable] -> Subsystem5/2(In2)
  [EMS_DecTar] -> Subsystem5/1(In1)
  Subsystem3/1(Function_Acc_status) -> Bus Creator/6  "Function_Acc_status"
  Bus Selector1/5 -> Data Type Conversion3/1  "<ACCSve_d_ACC_State_convert>"
  Subsystem2/1(StAcvTqWhlPTPotReq) -> Bus Creator/4  "StAcvTqWhlPTPotReq"
  [ESC_Enable] -> Subsystem2/2(In2)
  Subsystem1/1(TminUpGear) -> Bus Creator/3  "TminUpGear"
  Subsystem/1(TminDownGear) -> Bus Creator/2  "TminDownGear"
  [EMS_Enable] -> Subsystem1/1(In1), Subsystem/1(In1), Subsystem2/1(In1)
  ACT_Control_Signal/1 -> Bus Selector1/1
  Bus Creator/1 -> Signal Conversion/1
  [ESC_DecTar] -> Bus Creator/1  "Deceleration_setpoint_device"
  [EMS_DecTar] -> Gain/1, Bus Creator/7  "ACCTqReq"
  [ESC_Enable] -> Data Type Conversion1/1
  [ESC_Enable] -> Data Type Conversion2/1
  Data Type Conversion3/1 -> Subsystem3/1(In1)
  [ESC_Hold] -> Data Type Conversion5/1
  [ESC_EPB] -> Data Type Conversion6/1
  [ESC_DriveOff] -> Data Type Conversion4/1
  Bus Selector1/6 -> [ESC_DriveOff]  "<ACCSve_d_ACC_ESCDriveOff_convert>"
  Bus Selector1/7 -> [ESC_Hold]  "<ACCSve_d_ACC_ESCHoldReq_convert>"
  Bus Selector1/8 -> [ESC_EPB]  "<ACCSve_d_ACC_EPBReq_convert>"
  Data Type Conversion4/1 -> Bus Creator/13  "OMAPve_y_ADAS_ESCDriveOff"
  Data Type Conversion5/1 -> Bus Creator/14  "OMAPve_y_ADAS_ESCHoldReq"
  Data Type Conversion6/1 -> Bus Creator/15  "OMAPve_y_ADAS_ACCRequestEPB"

== system OMAP/Runnable_OMAP_10ms_sys/OMAP_Module/ACCS_Direct/ACCS_Define/Human_Machine_Interface(ACC_HMI)/Subsystem ==
  Distance : Inport
  CIPV_ID : Inport  Port=2
  ACC_State : Inport  Port=3
  Chart : Stateflow chart  TreatAsAtomicUnit=on
  Compare To Constant13 : simulink/Logic and Bit Operations/Compare To Constant  relop=>  const=0  OutDataTypeStr=boolean
  Compare To Constant14 : simulink/Logic and Bit Operations/Compare To Constant  relop===  const=4  OutDataTypeStr=boolean
  Compare To Constant16 : simulink/Logic and Bit Operations/Compare To Constant  relop===  const=7  OutDataTypeStr=boolean
  Compare To Constant17 : simulink/Logic and Bit Operations/Compare To Constant  relop===  const=8  OutDataTypeStr=boolean
  Compare To Constant18 : simulink/Logic and Bit Operations/Compare To Constant  relop===  const=5  OutDataTypeStr=boolean
  Constant : Constant  Value=5  OutDataTypeStr=uint8
  Constant1 : Constant  Value=0  OutDataTypeStr=uint8
  Logical Operator5 : Logic  Operator=OR  Inputs=4  AllPortsSameDT=off  OutDataTypeStr=boolean
  Switch : Switch  Criteria=u2 ~= 0
  Switch1 : Switch  Criteria=u2 ~= 0
  TARGET_POSITION : Outport
  TgDisp_Flag : Outport  Port=2
  wires:
  Distance/1 -> Chart/1(Distance)
  Chart/1(Value) -> Switch/1
  ACC_State/1 -> Compare To Constant16/1, Compare To Constant17/1, Compare To Constant14/1, Compare To Constant18/1
  Compare To Constant18/1 -> Logical Operator5/1
  Compare To Constant14/1 -> Logical Operator5/2
  Compare To Constant16/1 -> Logical Operator5/3
  Compare To Constant17/1 -> Logical Operator5/4
  Logical Operator5/1 -> Switch/2, Switch1/2
  Switch/1 -> TARGET_POSITION/1
  Constant/1 -> Switch/3
  Switch1/1 -> TgDisp_Flag/1
  CIPV_ID/1 -> Compare To Constant13/1
  Compare To Constant13/1 -> Switch1/1
  Constant1/1 -> Switch1/3

== system OMAP/Runnable_OMAP_10ms_sys/OMAP_Module/ACCS_Direct/ACCS_Define/Human_Machine_Interface(ACC_HMI)/Subsystem9 ==
  ACC_State : Inport
  ACCICA_Flag : Inport  Port=2
  VelocitySet : Inport  Port=3
  Bus Creator : BusCreator  Inputs=4
  Bus Selector : BusSelector  OutputSignals=ACC_Vehicle_Icon_Display,ACC_Set_Speed_Display,ACC_DesiredHeadway_Icon_Basic,RVVACC_Vehiclespeed_request_type
  Constant : Constant  Value=0  OutDataTypeStr=uint16
  Multiport Switch : MultiPortSwitch  DataPortOrder=Specify indices  DataPortIndices={0,1,2,3,4,5,6,7,8,15}  DiagnosticForDefault=Warning
  Subsystem : Subsystem
  Subsystem1 : Subsystem
  Subsystem2 : Subsystem
  Subsystem3 : Subsystem
  Subsystem4 : Subsystem
  Subsystem5 : Subsystem
  Subsystem6 : Subsystem
  Subsystem7 : Subsystem
  Subsystem8 : Subsystem
  Switch : Switch  Criteria=u2 ~= 0
  Out1 : Outport
  wires:
  Subsystem/1(Out1) -> Multiport Switch/2, Multiport Switch/3
  Multiport Switch/1 -> Bus Selector/1
  ACC_State/1 -> Multiport Switch/1
  Subsystem2/1(Out1) -> Multiport Switch/5
  Subsystem1/1(Out1) -> Multiport Switch/4
  Subsystem3/1(Out1) -> Multiport Switch/6
  Subsystem4/1(Out1) -> Multiport Switch/7
  Subsystem5/1(Out1) -> Multiport Switch/8
  Subsystem6/1(Out1) -> Multiport Switch/9
  Subsystem7/1(Out1) -> Multiport Switch/10
  Subsystem8/1(Out1) -> Multiport Switch/11
  VelocitySet/1 -> Subsystem2/1(VelocitySet), Subsystem1/1(VelocitySet)
  ACCICA_Flag/1 -> Switch/2
  Constant/1 -> Switch/1
  Bus Creator/1 -> Out1/1
  Bus Selector/1 -> Switch/3  "<ACC_Vehicle_Icon_Display>"
  Bus Selector/2 -> Bus Creator/2  "<ACC_Set_Speed_Display>"
  Bus Selector/3 -> Bus Creator/3  "<ACC_DesiredHeadway_Icon_Basic>"
  Bus Selector/4 -> Bus Creator/4  "<RVVACC_Vehiclespeed_request_type>"
  Switch/1 -> Bus Creator/1  "ACC_Vehicle_Icon_Display"

== system OMAP/Runnable_OMAP_10ms_sys/OMAP_Module/ACCS_Direct/ACCS_Define/Human_Machine_Interface(ACC_HMI)/Text_PopUp ==
  ACC_State : Inport
  ACCICA_Flag : Inport  Port=2
  ACCActive_Signal : Inport  Port=3
  go_request : Inport  Port=4
  ACC_DecReq : Inport  Port=5
  " Radar_Blocked" : Subsystem
  ACC_Activation_Unsatisfied : Subsystem
  ACC_Active : Subsystem
  ACC_Canceled : Subsystem
  ACC_Fault : Subsystem
  ACC_OFF : Subsystem
  ACC_ON : Subsystem
  ACC_go_request : Subsystem
  Cast : DataTypeConversion  OutDataTypeStr=uint8
  Constant : Constant  Value=0  OutDataTypeStr=uint16
  Constant1 : Constant  Value=0  OutDataTypeStr=uint16
  Gain : Gain
  Gain1 : Gain  Gain=10
  Gain2 : Gain  Gain=3
  Gain3 : Gain  Gain=8
  Gain4 : Gain  Gain=5
  Gain5 : Gain  Gain=2
  Gain6 : Gain  Gain=4
  Gain7 : Gain  Gain=7
  Gain9 : Gain  Gain=9
  Please_Take_Over_the_Car : Subsystem
  Please_Take_Over_the_Car_immediataly : Subsystem
  Radar_State : Constant  Value=2
  Switch{1..10} (10 alike) : Switch  Criteria=u2 > Threshold
  Switch11 : Switch  Criteria=u2 ~= 0
  Unit Delay1 : UnitDelay  SampleTime=-1
  gorequest : Gain  Gain=6
  For4F7 : Outport
  ForTJA : Outport  Port=2
  wires:
  ACC_ON/1(Out1) -> Gain/1
  Cast/1 -> " Radar_Blocked"/1(In1)
  " Radar_Blocked"/1(Out1) -> Gain5/1
  ACC_Fault/1(Out1) -> Gain2/1
  ACCActive_Signal/1 -> ACC_Activation_Unsatisfied/2(In2)
  ACC_Activation_Unsatisfied/1(Out1) -> Gain6/1
  ACC_Active/1(Out1) -> Gain4/1
  go_request/1 -> ACC_go_request/1(In1)
  ACC_go_request/1(<GoRequest>) -> gorequest/1
  Please_Take_Over_the_Car/1(Out1) -> Gain7/1
  ACC_State/1 -> ACC_OFF/1(In1), ACC_Canceled/1(In1), Please_Take_Over_the_Car/1(In1), ACC_Active/1(In1), ACC_Activation_Unsatisfied/1(In1), ACC_Fault/1(In1), ACC_ON/1(In1)
  Please_Take_Over_the_Car_immediataly/1(Out1) -> Gain3/1
  ACC_Canceled/1(Out1) -> Gain9/1
  ACC_OFF/1(Out1) -> Gain1/1
  Gain/1 -> Switch1/1, Switch1/2
  Gain5/1 -> Switch2/1, Switch2/2
  Gain2/1 -> Switch3/1, Switch3/2
  Gain6/1 -> Switch4/1, Switch4/2
  Gain4/1 -> Switch5/1, Switch5/2
  gorequest/1 -> Switch6/1, Switch6/2
  Gain7/1 -> Switch7/1, Switch7/2
  Gain3/1 -> Switch8/1, Switch8/2
  Gain9/1 -> Switch9/1, Switch9/2
  Constant/1 -> Switch1/3
  Switch1/1 -> Switch2/3
  Switch2/1 -> Switch3/3
  Switch3/1 -> Switch4/3
  Switch4/1 -> Switch5/3
  Switch5/1 -> Switch6/3
  Switch6/1 -> Switch7/3
  Switch7/1 -> Switch8/3
  Switch8/1 -> Switch9/3
  Gain1/1 -> Switch10/1, Switch10/2
  Switch9/1 -> Switch10/3
  Switch10/1 -> Unit Delay1/1, ForTJA/1, Switch11/3
  [ACCICA_Flag] -> Switch11/2
  Constant1/1 -> Switch11/1
  Switch11/1 -> For4F7/1
  [Text] -> ACC_ON/2(In2)
  Unit Delay1/1 -> [Text]
  [ACCICA_Flag] -> ACC_OFF/2(In2)
  ACCICA_Flag/1 -> [ACCICA_Flag]
  [ACCICA_Flag] -> ACC_ON/3(ACCICA_Flag)
  Radar_State/1 -> Cast/1
  ACC_DecReq/1 -> Please_Take_Over_the_Car_immediataly/1(ESC_DecTar)

== system OMAP/Runnable_OMAP_10ms_sys/OMAP_Module/ICA_Direct_G59/ICA_Define/ICA_EPS/EPS_Ctr_Disable ==
  note: 默认值2
  stEPSCtlState : Inport
  Action Port : ActionPort  InitializeStates=reset  ActionType=else
  Constant : Constant  Value=0  OutDataTypeStr=single
  Constant1 : Constant  Value=0  OutDataTypeStr=uint16
  Constant2 : Constant  Value=OMAP_ICA_EPSCMDdisable  OutDataTypeStr=uint8
  Constant3 : Constant  Value=0  OutDataTypeStr=single
  Constant4 : Constant  Value=0  OutDataTypeStr=single
  MATLAB Function : MATLAB Function  TreatAsAtomicUnit=on
  stEPSCtlCMD : Outport
  LKA_TRQ_FACT_REQ : Outport  Port=2
  LKA_OR_LPA_REQ : Outport  Port=3
  angle1 : Outport  Port=4
  torque1 : Outport  Port=5
  wires:
  MATLAB Function/1(stEPSCtlCMD) -> stEPSCtlCMD/1
  stEPSCtlState/1 -> MATLAB Function/1(stEPSCtlState)
  Constant/1 -> LKA_TRQ_FACT_REQ/1  "LKA_TRQ_FACT_REQ"
  Constant1/1 -> LKA_OR_LPA_REQ/1  "LKA_OR_LPA_REQ"
  Constant3/1 -> angle1/1  "LKA_OR_LPA_REQ"
  Constant4/1 -> torque1/1  "LKA_OR_LPA_REQ"
  Constant2/1 -> MATLAB Function/2(ControlCMDdisable)

== system OMAP/Runnable_OMAP_10ms_sys/OMAP_Module/ICA_Direct_G59/ICA_Define/ICA_EPS/EPS_Ctr_Enable ==
  note: 默认值2
  note: 默认值3
  note: 默认值4
  stEPSCtlState : Inport
  angle : Inport  Port=2
  torque : Inport  Port=3
  Action Port : ActionPort  InitializeStates=reset  ActionType=then
  Abs : Abs
  Constant : Constant  Value=OMAP_ICA_EPStrqfactor  OutDataTypeStr=single
  Constant1 : Constant  Value=0  OutDataTypeStr=uint16
  Constant2 : Constant  Value=OMAP_ICA_EPSCMDselect  OutDataTypeStr=uint8
  Constant3 : Constant  Value=OMAP_ICA_EPSCMDauthorized  OutDataTypeStr=uint8
  Constant4 : Constant  Value=OMAP_ICA_EPSCMDactive  OutDataTypeStr=uint8
  Constant5 : Constant  Value=OMAP_ICA_EPStrqfactorRate  OutDataTypeStr=single
  Gain : Gain  Gain=-1  OutDataTypeStr=single
  MATLAB Function : MATLAB Function  TreatAsAtomicUnit=on
  Rate Limiter Dynamic : simulink/Discontinuities/Rate Limiter Dynamic
      settings: SourceProductName=Simulink
  stEPSCtlCMD : Outport
  LKA_TRQ_FACT_REQ : Outport  Port=2
  LKA_OR_LPA_REQ : Outport  Port=3
  angle1 : Outport  Port=4
  torque1 : Outport  Port=5
  wires:
  stEPSCtlState/1 -> MATLAB Function/1(stEPSCtlState)
  MATLAB Function/1(stEPSCtlCMD) -> stEPSCtlCMD/1
  Rate Limiter Dynamic/1 -> LKA_TRQ_FACT_REQ/1  "LKA_TRQ_FACT_REQ"
  Constant1/1 -> LKA_OR_LPA_REQ/1  "LKA_OR_LPA_REQ"
  angle/1 -> angle1/1
  torque/1 -> torque1/1
  Constant2/1 -> MATLAB Function/2(EPSCMDselect)
  Constant3/1 -> MATLAB Function/3(EPSCMDauthorized)
  Constant4/1 -> MATLAB Function/4(EPSCMDactive)
  Constant/1 -> Rate Limiter Dynamic/2  "LKA_TRQ_FACT_REQ"
  Constant5/1 -> Abs/1  "LKA_TRQ_FACT_REQ"
  Abs/1 -> Gain/1, Rate Limiter Dynamic/1
  Gain/1 -> Rate Limiter Dynamic/3
